simulink model "pendulo_invertido"  (R2026a)
settings: Solver=ode45  StopTime=t_final
InitFcn:
  | run('/home/sergio/Escritorio/tdc/proyecto-1-pendulo-invertido/init_pendulo_simulink.m')
values from neighbouring files (symbols this model uses):
  K_lqr = lqr_data.K    [init_pendulo_simulink.m]
  umax = p.umax    [init_pendulo_simulink.m]
  x0_sim = p.x0_default    [init_pendulo_simulink.m]
undefined symbols (not defined in the file or in its folder): A_lin, B_lin, C_lin, D_lin
settings Model: Creator=sergio  LastModifiedBy=sergio
settings DataIOCC: SaveFormat=StructureWithTime

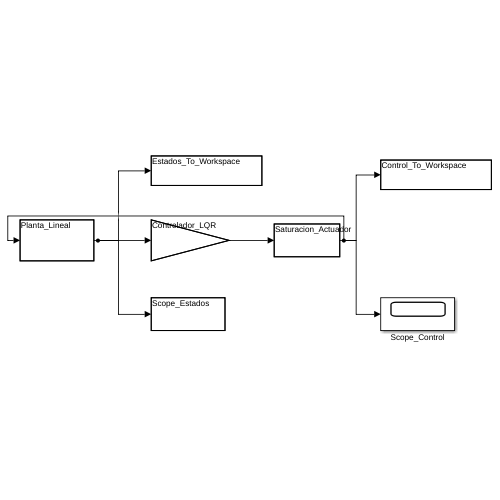
[thumbnail: Simulink's stored preview of the top-level diagram]
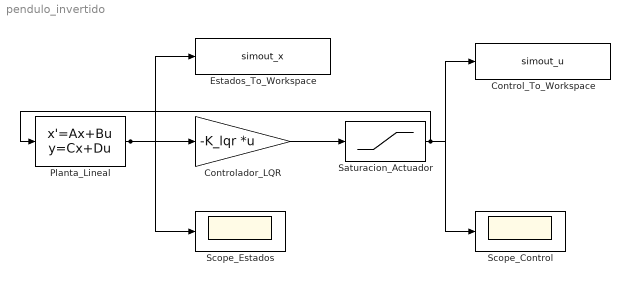
== system pendulo_invertido ==
  Control_To_Workspace : ToWorkspace  VariableName=simout_u  SaveFormat=Structure With Time  SampleTime=-1
  Controlador_LQR : Gain  Gain=-K_lqr  Multiplication=Matrix(K*u)
  Estados_To_Workspace : ToWorkspace  VariableName=simout_x  SaveFormat=Structure With Time  SampleTime=-1
  Planta_Lineal : StateSpace  A=A_lin  B=B_lin  C=C_lin  D=D_lin  InitialCondition=x0_sim
  Saturacion_Actuador : Saturate  UpperLimit=umax  LowerLimit=-umax
  Scope_Control : Scope
  Scope_Estados : Scope
  wires:
  Planta_Lineal/1 -> Controlador_LQR/1, Estados_To_Workspace/1, Scope_Estados/1
  Controlador_LQR/1 -> Saturacion_Actuador/1
  Saturacion_Actuador/1 -> Planta_Lineal/1, Control_To_Workspace/1, Scope_Control/1
